simulink model "GuytonModel1986All_R2015a"  (R2015a)
settings: Solver=ode15s  StartTime=0  StopTime=383040  FixedStep=0.03  MaxStep=360  RelTol=1e-3
libraries: simulink x3
(part 2 of 5)

== system GuytonModel1986All_R2015a/Afferent Arteriole ==
  note: AFFERENT ARTERIOLE
  note: RNAUG1
  note: AUMK
  AARK : Inport
  MYOGRSAA : Inport  Port=2
  RNAUG1 : Inport  Port=3
  ANM : Inport  Port=4
  AUM : Inport  Port=5
  VIM : Inport  Port=6
  ANMAM : Constant  Value=0.5
  ANMAM1 : Constant
  ANMAM2 : Constant
  ARF : Constant  Value=1.5
  Constant1 : Constant
  Constant35 : Constant
  Product1 : Product  SaturateOnIntegerOverflow=on  RndMeth=Zero  InputSameDT=on  OutDataTypeStr=Inherit: Same as first input
  Product11 : Product  SaturateOnIntegerOverflow=on  RndMeth=Zero  InputSameDT=on  OutDataTypeStr=Inherit: Same as first input
  Product12 : Product  Inputs=6  SaturateOnIntegerOverflow=on  RndMeth=Zero  InputSameDT=on  OutDataTypeStr=Inherit: Same as first input
  Sum1 : Sum  SaturateOnIntegerOverflow=on  InputSameDT=on  OutDataTypeStr=Inherit: Same as first input
  Sum18 : Sum  Inputs=+-  SaturateOnIntegerOverflow=on  InputSameDT=on  OutDataTypeStr=Inherit: Same as first input
  Sum2 : Sum  Inputs=+-  SaturateOnIntegerOverflow=on  InputSameDT=on  OutDataTypeStr=Inherit: Same as first input
  Sum3 : Sum  SaturateOnIntegerOverflow=on  InputSameDT=on  OutDataTypeStr=Inherit: Same as first input
  lower limit 0.8 : Saturate  UpperLimit=inf  LowerLimit=0.86
  lower limit 0.86 : Saturate  UpperLimit=inf  LowerLimit=0.86
  lower limit 18 : Saturate  UpperLimit=inf  LowerLimit=18
  AAR : Outport
  wires:
  ANM/1 -> Sum18/1
  Constant35/1 -> Sum18/2
  ANMAM/1 -> Product11/2
  Sum18/1 -> Product11/1
  Product12/1 -> lower limit 18/1
  lower limit 18/1 -> AAR/1
  Product11/1 -> Sum1/1
  ANMAM1/1 -> Sum1/2
  Sum1/1 -> lower limit 0.86/1
  AARK/1 -> Product12/1  "AARK"
  MYOGRSAA/1 -> Product12/2  "MYOGRSAA"
  RNAUG1/1 -> Product12/3
  VIM/1 -> Product12/4  "VIM"
  lower limit 0.86/1 -> Product12/6  "ANIM"
  AUM/1 -> Sum2/1
  Constant1/1 -> Sum2/2
  Sum2/1 -> Product1/1
  ARF/1 -> Product1/2
  Product1/1 -> Sum3/1
  ANMAM2/1 -> Sum3/2
  Sum3/1 -> lower limit 0.8/1
  lower limit 0.8/1 -> Product12/5

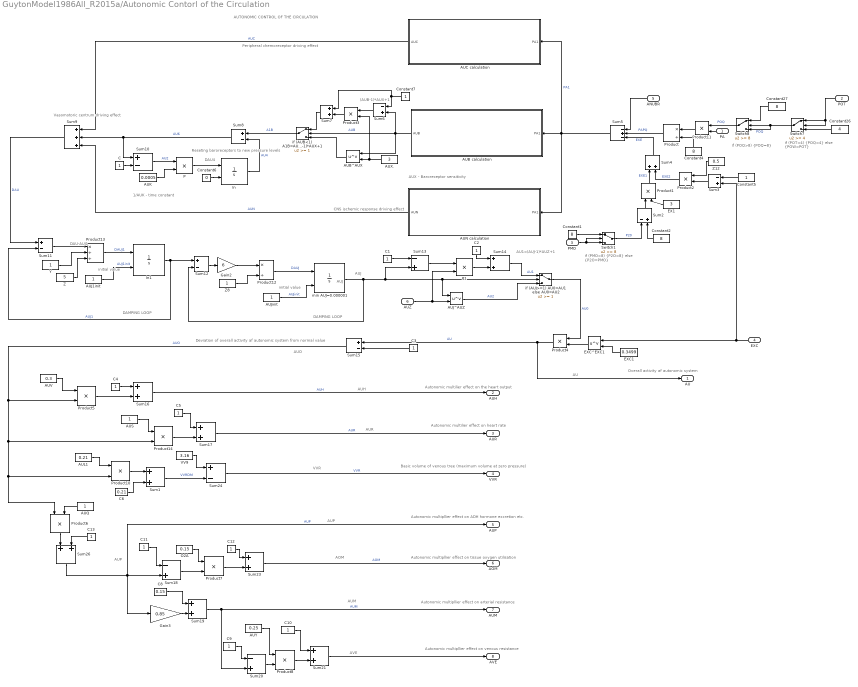
== system GuytonModel1986All_R2015a/Autonomic Contorl of the Circulation ==
  note: AUTONOMIC CONTROL OF THE CIRCULATION
  note: Autonomic multipllier effect on venous resistance
  note: Autonomic multipllier effect on arterial resistance
  note: Basic volume of venous tree (maximum volume at zero pressure)
  note: Autonomic multilier effect on heart rate
  note: Autonomic multipllier effect on tissue oxygen utilisation
  note: Autonomic multipllier effect on ADH hormone excretion etc.
  note: Autonomic multilier effect on the heart output
  note: Deviation of overall activity af autonomic system from normal value
  note: AUO
  note: Overall activity af autonomic system
  note: AU
  note: AU1=(AUJ-1)*AUZ+1
  note: initial value
  note: AUJ
  note: DAMPING LOOP
  note: DAMPING LOOP
  note: initial value
  note: AUJ
  note: DAU-AUJ1
  note: 1/AUK - time constant
  note: CNS ischemic response driving effect
  note: Vasomotoric centrum driving effect
  note: Peripheral chemoreceptor driving effect
  note: Reseting baroreceptors to new pressure levels
  note: DAU4
  note: AUX - Baroreceptor sensitivity
  note: (AUB-1)*AUX+1
  note: if (PMO>8)  {P2O=8}
      | else {P2O=PMO}
  note: if (POQ>8) {POQ=8}
  note: if (POT<4) {POQ=4}
      | else {POW=POT}
  note: AOM
  note: AUP
  note: AVE
  note: AUM
  note: VVR
  note: AUP
  note: AUR
  note: AUH
  PA : Inport
  POT : Inport  Port=2
  PMO : Inport  Port=3
  EXC : Inport  Port=4
  ANUBR : Inport  Port=5
  AUZ : Inport  Port=6
  AUB calculation : Subsystem
      mask Display: disp('AUB CALCULATION \n\nwhen PA1<40: AUB=1.85718             \nwhen  40>PA1<170: AUB=0.014286*(170-PA1)\nwhen PA1>=170: AUB=0               \n')
  AUB^AUX : Math  Operator=pow  SaturateOnIntegerOverflow=on
  AUC calculation : Subsystem
      mask Display: disp('AUC CALCULATION \n\nwhen PA1<40: AUC=1.2             \nwhen  40>PA1<80: AUC=0.03*(80-PA1)\nwhen PA1>=80: AUC=0               \n')
  AUJ1init : Constant
  AUJ^AUZ : Math  Operator=pow  SaturateOnIntegerOverflow=on
  AUJinit : Constant
  AUK : Constant  Value=0.0005
  AUL1 : Constant  Value=0.21
  AUN calculation : Subsystem
      mask Display: disp('AUN CALCULATION \n\nwhen PA1<50: AUN=6             \nwhen  20>PA1<50: AUN=0.2*(50-PA1)\nwhen PA1>=50: AUC=0               \n')
  AUQ : Constant
  AUS : Constant
  AUV : Constant  Value=0.3
  AUX. : Constant  Value=3
  AUY : Constant  Value=0.25
  C{,1..5,9..13} (11 alike) : Constant
  C6 : Constant  Value=0.21
  C8 : Constant  Value=0.15
  Constant{1..2,4,27} (4 alike) : Constant  Value=8
  Constant26 : Constant  Value=4
  Constant5 : Constant
  Constant6 : Constant  Value=0
  Constant7 : Constant
  EX1 : Constant  Value=3
  EXC1 : Constant  Value=0.3499
  EXC^EXC1 : Math  Operator=pow  SaturateOnIntegerOverflow=on
  Gain2 : Gain  Gain=6  SaturateOnIntegerOverflow=on  OutDataTypeStr=Inherit: Same as input  ParamDataTypeStr=Inherit: Same as input
  Gain3 : Gain  Gain=0.85  SaturateOnIntegerOverflow=on  OutDataTypeStr=Inherit: Same as input  ParamDataTypeStr=Inherit: Same as input
  In : Integrator  InitialConditionSource=external  InitialCondition=0.012127
  In1 : Integrator  InitialConditionSource=external  InitialCondition=1
  O2A : Constant  Value=0.15
  P : Product  SaturateOnIntegerOverflow=on  RndMeth=Zero  InputSameDT=on  OutDataTypeStr=Inherit: Same as first input
  P1 : Product  SaturateOnIntegerOverflow=on  RndMeth=Zero  InputSameDT=on  OutDataTypeStr=Inherit: Same as first input
  Product : Product  Inputs=*/  SaturateOnIntegerOverflow=on  RndMeth=Zero  InputSameDT=on  OutDataTypeStr=Inherit: Same as first input
  Product{1..8,10..11,14} (11 alike) : Product  SaturateOnIntegerOverflow=on  RndMeth=Zero  InputSameDT=on  OutDataTypeStr=Inherit: Same as first input
  Product12 : Product  Inputs=*/  SaturateOnIntegerOverflow=on  RndMeth=Zero  InputSameDT=on  OutDataTypeStr=Inherit: Same as first input
  Product13 : Product  Inputs=*//  SaturateOnIntegerOverflow=on  RndMeth=Zero  InputSameDT=on  OutDataTypeStr=Inherit: Same as first input
  Sum{1,4,7,14,16..17,19,21,23,26} (10 alike) : Sum  SaturateOnIntegerOverflow=on  InputSameDT=on  OutDataTypeStr=Inherit: Same as first input
  Sum{8,10..12,15,24} (6 alike) : Sum  Inputs=+-  SaturateOnIntegerOverflow=on  InputSameDT=on  OutDataTypeStr=Inherit: Same as first input
  Sum{2..3,6,13,18,20} (6 alike) : Sum  Inputs=-+  SaturateOnIntegerOverflow=on  InputSameDT=on  OutDataTypeStr=Inherit: Same as first input
  Sum5 : Sum  Inputs=-+-  SaturateOnIntegerOverflow=on  InputSameDT=on  OutDataTypeStr=Inherit: Same as first input
  Sum9 : Sum  Inputs=+++  SaturateOnIntegerOverflow=on  InputSameDT=on  OutDataTypeStr=Inherit: Same as first input
  Switch1 : Switch  Threshold=8  SaturateOnIntegerOverflow=on  InputSameDT=on
  Switch7 : Switch  Threshold=4  SaturateOnIntegerOverflow=on  InputSameDT=on
  Switch8 : Switch  Threshold=8  SaturateOnIntegerOverflow=on  InputSameDT=on
  VV9 : Constant  Value=3.16
  Y : Constant
  Z : Constant  Value=5
  Z12 : Constant  Value=0.5
  Z8 : Constant
  if (AUB<1) A1B=AUB^AUX else A1B=(AUB-1)*AUX+1 : Switch  Threshold=1  SaturateOnIntegerOverflow=on  InputSameDT=on
  if (AUJ>=1) AU0=AU1 else AU0=AU2 : Switch  Threshold=1  SaturateOnIntegerOverflow=on  InputSameDT=on
  min AUJ=0.000001 : Integrator  InitialConditionSource=external  InitialCondition=1  LimitOutput=on  LowerSaturationLimit=0
  AU : Outport
  AUH : Outport  Port=2
  AUR : Outport  Port=3
  VVR : Outport  Port=4
  AUP : Outport  Port=5
  AOM : Outport  Port=6
  AUM : Outport  Port=7
  AVE : Outport  Port=8
  wires:
  Constant6/1 -> In/2
  Sum21/1 -> AVE/1
  C10/1 -> Sum21/1
  Product8/1 -> Sum21/2
  AUY/1 -> Product8/1
  Sum20/1 -> Product8/2
  Sum1/1 -> Sum24/2  "VVRDM"
  Product10/1 -> Sum1/1
  C6/1 -> Sum1/2
  Sum24/1 -> VVR/1  "VVR"
  VV9/1 -> Sum24/1
  AUL1/1 -> Product10/1
  C13/1 -> Sum26/2
  Product6/1 -> Sum26/1
  EXC^EXC1/1 -> Product4/2
  EXC1/1 -> EXC^EXC1/2
  C1/1 -> Sum13/1
  Sum13/1 -> P1/1
  AUJinit/1 -> min AUJ=0.000001/2  "AUJinit"
  AUJ1init/1 -> In1/2  "AUJ1init"
  In1/1 -> Sum11/2, Sum12/1  "AUJ1"
  AUX./1 -> Product3/2, AUB^AUX/2
  AUB^AUX/1 -> if (AUB<1) A1B=AUB^AUX else A1B=(AUB-1)*AUX+1/3
  Sum7/1 -> if (AUB<1) A1B=AUB^AUX else A1B=(AUB-1)*AUX+1/1
  Product3/1 -> Sum7/2
  Sum6/1 -> Product3/1
  Constant7/1 -> Sum6/1, Sum7/1
  AUB calculation/1(AUB) -> AUB^AUX/1, Sum6/2, if (AUB<1) A1B=AUB^AUX else A1B=(AUB-1)*AUX+1/2  "AUB"
  Switch1/1 -> Sum2/1  "P20"
  PMO/1 -> Switch1/3, Switch1/2
  Constant1/1 -> Switch1/1
  EXC/1 -> EXC^EXC1/1, Sum3/2
  Switch8/1 -> Product11/1  "POQ"
  Constant27/1 -> Switch8/1
  Switch7/1 -> Switch8/3, Switch8/2  "POQ"
  Constant26/1 -> Switch7/3
  Product11/1 -> Product/1
  Product/1 -> Sum5/2  "PAPQ"
  C12/1 -> Sum23/1
  Product7/1 -> Sum23/2
  O2A/1 -> Product7/1
  Sum18/1 -> Product7/2
  C11/1 -> Sum18/1
  Sum19/1 -> AUM/1, Sum20/2  "AUM"
  C9/1 -> Sum20/1
  C8/1 -> Sum19/1
  Gain3/1 -> Sum19/2
  Sum26/1 -> Gain3/1, Sum18/2, AUP/1  "AUP"
  AUQ/1 -> Product6/2
  Sum17/1 -> AUR/1  "AUR"
  C5/1 -> Sum17/1
  Product14/1 -> Sum17/2
  AUS/1 -> Product14/1
  C4/1 -> Sum16/1
  Product5/1 -> Sum16/2
  AUV/1 -> Product5/1
  C3/1 -> Sum15/2
  Product4/1 -> Sum15/1, AU/1  "AU"
  Sum14/1 -> if (AUJ>=1) AU0=AU1 else AU0=AU2/1  "AU1"
  C2/1 -> Sum14/1
  P1/1 -> Sum14/2
  AUJ^AUZ/1 -> if (AUJ>=1) AU0=AU1 else AU0=AU2/3  "AU2"
  min AUJ=0.000001/1 -> Sum12/2, AUJ^AUZ/1, if (AUJ>=1) AU0=AU1 else AU0=AU2/2, Sum13/2
  Product12/1 -> min AUJ=0.000001/1  "DAUJ"
  Gain2/1 -> Product12/1
  Sum12/1 -> Gain2/1
  Y/1 -> Product13/2
  P/1 -> In/1
  AUK/1 -> P/2
  Sum10/1 -> P/1  "AU2"
  C/1 -> Sum10/2
  Sum8/1 -> Sum9/2, Sum10/1  "AU6"
  ANUBR/1 -> Sum5/1
  Product1/1 -> Sum4/1  "EXE1"
  Product2/1 -> Sum4/2  "EXE2"
  Z12/1 -> Product2/1
  Sum3/1 -> Product2/2
  Constant5/1 -> Sum3/1
  EX1/1 -> Product1/2
  Sum2/1 -> Product1/1
  Constant2/1 -> Sum2/2
  AUZ/1 -> P1/2, AUJ^AUZ/2
  Sum4/1 -> Sum5/3  "EXE"
  POT/1 -> Switch7/1, Switch7/2
  Constant4/1 -> Product/2
  PA/1 -> Product11/2
  Sum5/1 -> AUN calculation/1(PA1), AUB calculation/1(PA1), AUC calculation/1(PA1)  "PA1"
  AUN calculation/1(AUN) -> Sum9/3  "AUN"
  AUC calculation/1(AUC) -> Sum9/1  "AUC"
  if (AUB<1) A1B=AUB^AUX else A1B=(AUB-1)*AUX+1/1 -> Sum8/1  "A1B"
  In/1 -> Sum8/2  "AU4"
  Sum9/1 -> Sum11/1  "DAU"
  Z/1 -> Product13/3
  Product13/1 -> In1/1  "DAUJ1"
  Sum11/1 -> Product13/1
  Z8/1 -> Product12/2
  if (AUJ>=1) AU0=AU1 else AU0=AU2/1 -> Product4/1  "AU0"
  Sum15/1 -> Product10/2, Product6/1, Product14/2, Product5/2  "AUO"
  Sum23/1 -> AOM/1  "AOM"
  Sum16/1 -> AUH/1  "AUH"

== system GuytonModel1986All_R2015a/Blood viscosity ==
  note: HM
  note: VIM
  note: Blood viscosity
  HM : Inport
  Constant1 : Constant  Value=3
  Constant7 : Constant  Value=1.5
  HKM : Constant  Value=0.53333
  HMK : Constant  Value=90
  Product1 : Product  Inputs=*/  SaturateOnIntegerOverflow=on  RndMeth=Zero  InputSameDT=on  OutDataTypeStr=Inherit: Same as first input
  Product7 : Product  Inputs=*/  SaturateOnIntegerOverflow=on  RndMeth=Zero  InputSameDT=on  OutDataTypeStr=Inherit: Same as first input
  Product8 : Product  Inputs=*/  SaturateOnIntegerOverflow=on  RndMeth=Zero  InputSameDT=on  OutDataTypeStr=Inherit: Same as first input
  Sum8 : Sum  Inputs=+-  SaturateOnIntegerOverflow=on  InputSameDT=on  OutDataTypeStr=Inherit: Same as first input
  Sum9 : Sum  SaturateOnIntegerOverflow=on  InputSameDT=on  OutDataTypeStr=Inherit: Same as first input
  VIM : Outport
  wires:
  Constant1/1 -> Product1/2
  Product1/1 -> VIM/1
  HM/1 -> Product7/1, Sum8/2  "HM"
  HMK/1 -> Sum8/1
  Sum8/1 -> Product7/2
  Product7/1 -> Product8/1
  HKM/1 -> Product8/2
  Product8/1 -> Sum9/1  "VIE"
  Constant7/1 -> Sum9/2
  Sum9/1 -> Product1/1  "VIB"

== system GuytonModel1986All_R2015a/Capillary Membrane Fluid Dynamics ==
  note: Capillary Membrane Fluid Dynamics
  PC : Inport
  PPC : Inport  Port=2
  PGH : Inport  Port=3
  PTC : Inport  Port=4
  VTL : Inport  Port=5
  TVD : Inport  Port=6
  VUD : Inport  Port=7
  DFP : Inport  Port=8
  VID : Inport  Port=9
  CFC : Inport  Port=10
  VPN : Inport  Port=11
  VTSN : Inport  Port=12
  Add : Sum
  Add1 : Sum  Inputs=-+
  CPK : Constant  Value=0.000253
  Integrator : Integrator  InitialConditionSource=external
  Integrator1 : Integrator  InitialConditionSource=external
  Math Function : Math  Operator=pow  SaturateOnIntegerOverflow=on
  PCE : Constant  Value=1.000
  PCR : Constant  Value=15
  PCR1 : Constant  Value=0
  Product : Product  RndMeth=Zero
  Product1 : Product  RndMeth=Zero
  Product2 : Product  Inputs=*/  RndMeth=Zero
  Product3 : Product  Inputs=*/  RndMeth=Zero
  Sum1 : Sum  Inputs=-++--  SaturateOnIntegerOverflow=on  InputSameDT=on  OutDataTypeStr=Inherit: Same as first input
  Sum2 : Sum  Inputs=-+-  SaturateOnIntegerOverflow=on  InputSameDT=on  OutDataTypeStr=Inherit: Same as first input
  Sum3 : Sum  Inputs=+--+  SaturateOnIntegerOverflow=on  InputSameDT=on  OutDataTypeStr=Inherit: Same as first input
  "if (PCRD1<0)  {PCRD=0} else {PCRD=PCRD1}" : Switch
  VP : Outport
  VTCLP : Outport  Port=2
  VTS : Outport  Port=3
  CFILTR : Outport  Port=4
  VTC : Outport  Port=5
  VPREL : Outport  Port=6
  VTSREL : Outport  Port=7
  wires:
  PC/1 -> Sum3/1, Add1/2
  PPC/1 -> Sum3/2
  PGH/1 -> Sum3/3
  PTC/1 -> Sum3/4
  Sum3/1 -> Product/1  "PCGR"
  CFC/1 -> Product/2
  Product/1 -> Add/2, CFILTR/1  "CFILTR"
  PCR/1 -> Add1/1
  Add1/1 -> "if (PCRD1<0)  {PCRD=0} else {PCRD=PCRD1}"/2, "if (PCRD1<0)  {PCRD=0} else {PCRD=PCRD1}"/1  "PCRD1"
  PCR1/1 -> "if (PCRD1<0)  {PCRD=0} else {PCRD=PCRD1}"/3
  "if (PCRD1<0)  {PCRD=0} else {PCRD=PCRD1}"/1 -> Product1/2  "PCRD"
  CPK/1 -> Product1/1
  Math Function/1 -> Add/1, VTCLP/1  "VTCPL"
  Add/1 -> Sum2/2, Sum1/1, VTC/1  "VTC"
  VTL/1 -> Sum1/2, Sum2/1
  TVD/1 -> Sum1/3
  VUD/1 -> Sum1/4
  DFP/1 -> Sum1/5
  Sum1/1 -> Integrator/1  "VPD"
  VTSN/1 -> Integrator1/2, Product3/2
  Sum2/1 -> Integrator1/1  "VTS"
  VID/1 -> Sum2/3
  Integrator/1 -> VP/1, Product2/1  "VP"
  Integrator1/1 -> VTS/1, Product3/1  "VTS"
  Product1/1 -> Math Function/1  "U"
  PCE/1 -> Math Function/2  "v"
  VPN/1 -> Integrator/2, Product2/2
  Product2/1 -> VPREL/1
  Product3/1 -> VTSREL/1

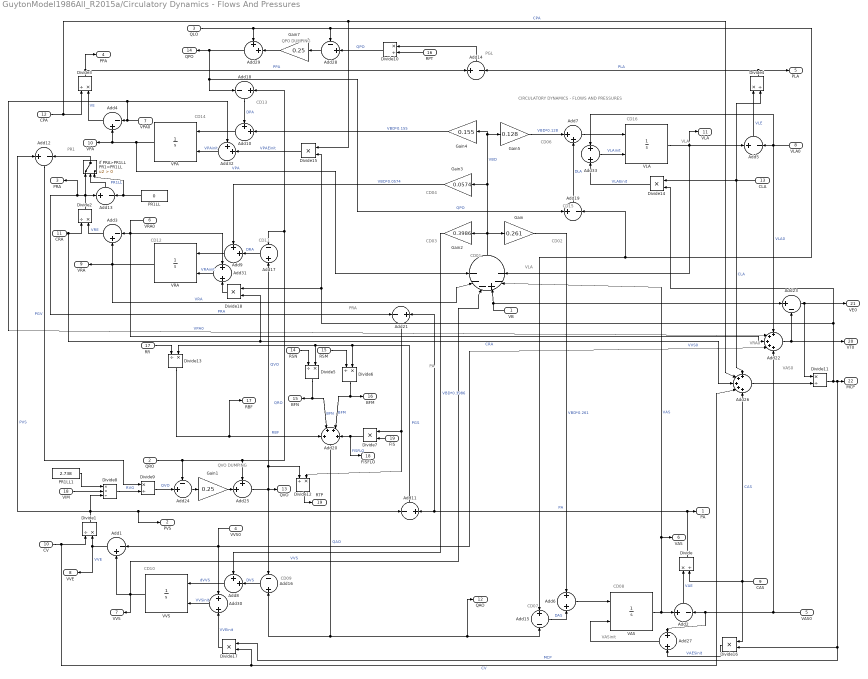
== system GuytonModel1986All_R2015a/Circulatory Dynamics - Flows And Pressures ==
  note: CD16
  note: CD15
  note: CD14
  note: CD12
  note: CD11
  note: CD10
  note: CD09
  note: CD08
  note: CD07
  note: CD06
  note: CD13
  note: CD04
  note: CD03
  note: CD02
  note: CD01
  note: CIRCULATORY DYNAMICS - FLOWS AND PRESSURES
  note: VAS0
  note: VRA0
  note: VASinit
  note: PRA
  note: PA
  note: PGL
  note: PR1
  note: VLA
  note: VLA
  note: QVO DUMPING
  note: QPO DUMPING
  VB : Inport
  QRO : Inport  Port=2
  QLO : Inport  Port=3
  VVS0 : Inport  Port=4
  VAS0 : Inport  Port=5
  VRA0 : Inport  Port=6
  VPA0 : Inport  Port=7
  VLA0 : Inport  Port=8
  CAS : Inport  Port=9
  CV : Inport  Port=10
  CRA : Inport  Port=11
  CPA : Inport  Port=12
  CLA : Inport  Port=13
  RSN : Inport  Port=14
  RSM : Inport  Port=15
  RPT : Inport  Port=16
  RR : Inport  Port=17
  VIM : Inport  Port=18
  FIS : Inport  Port=19
  " " : Sum  Inputs=---+--
  " VAS" : Integrator  InitialConditionSource=external
  " VLA" : Integrator  InitialConditionSource=external
  " VPA" : Integrator  InitialConditionSource=external
  " VRA" : Integrator  InitialConditionSource=external
  " VVS" : Integrator  InitialConditionSource=external
  Add1 : Sum  Inputs=|-+
  Add{8..10,25,29,32} (6 alike) : Sum  Inputs=++|
  Add{11,16..18,21} (5 alike) : Sum  Inputs=-+
  Add{2,5,12..15,19} (7 alike) : Sum  Inputs=+-
  Add20 : Sum  Inputs=++++
  Add22 : Sum  Inputs=5
  Add23 : Sum  Inputs=|+-
  Add24 : Sum  Inputs=-+|
  Add26 : Sum  Inputs=5
  Add{6,27,30..31,33} (5 alike) : Sum
  Add28 : Sum  Inputs=-+|
  Add3 : Sum  Inputs=|-+
  Add4 : Sum  Inputs=|-+
  Add7 : Sum  Inputs=|++
  Divide{,4,9..11} (5 alike) : Product  Inputs=*/
  Divide{1..3,5..6,12..13} (7 alike) : Product  Inputs=/*
  Divide{7,14..18} (6 alike) : Product  Inputs=**
  Divide8 : Product  Inputs=**/
  Gain : Gain  Gain=0.261
  Gain1 : Gain  Gain=0.25
  Gain2 : Gain  Gain=0.3986
  Gain3 : Gain  Gain=0.0574
  Gain4 : Gain  Gain=0.155
  Gain5 : Gain  Gain=0.128
  Gain7 : Gain  Gain=0.25
  PR1LL : Constant  Value=0
  PR1LL1 : Constant  Value=2.738
  if PRA>PR1LL PR1=PR1LL : Switch  Criteria=u2 > Threshold
  PA : Outport
  PVS : Outport  Port=2
  PRA : Outport  Port=3
  PPA : Outport  Port=4
  PLA : Outport  Port=5
  VAS : Outport  Port=6
  VVS : Outport  Port=7
  VVE : Outport  Port=8
  VRA : Outport  Port=9
  VPA : Outport  Port=10
  VLA : Outport  Port=11
  QAO : Outport  Port=12
  QVO : Outport  Port=13
  QPO : Outport  Port=14
  BFN : Outport  Port=15
  BFM : Outport  Port=16
  RBF : Outport  Port=17
  FISFLO : Outport  Port=18
  RTP : Outport  Port=19
  VT0 : Outport  Port=20
  VE0 : Outport  Port=21
  MCP : Outport  Port=22
  wires:
  Add33/1 -> " VLA"/2  "VLAinit"
  Divide15/1 -> Add32/2  "VPAEinit"
  Add32/1 -> " VPA"/2  "VPAinit"
  Divide18/1 -> Add31/2
  Add31/1 -> " VRA"/2  "VRAinit"
  Divide17/1 -> Add30/2  "VVEinit"
  Add30/1 -> " VVS"/2  "VVSinit"
  VVS0/1 -> Add22/4, Add1/1, Add30/1  "VVS0"
  Add27/1 -> " VAS"/2
  Divide16/1 -> Add27/2  "VAESinit"
  Divide14/1 -> Add33/2  "VLAEinit"
  Divide11/1 -> Divide17/1, Divide16/2, MCP/1, Divide15/2, Divide18/1, Divide14/2  "MCP"
  Add26/1 -> Divide11/2
  Divide13/1 -> Add20/1, RBF/1  "RBF"
  RR/1 -> Divide13/1
  Add6/1 -> " VAS"/1
  " "/1 -> Gain5/1, Gain4/1, Gain3/1, Gain2/1, Gain/1  "VBD"
  Add23/1 -> Divide11/1, VE0/1
  Add22/1 -> Add23/2, VT0/1
  if PRA>PR1LL PR1=PR1LL/1 -> Add12/2
  Add5/1 -> Divide4/1  "VLE"
  Add4/1 -> Divide3/2  "VE"
  Divide12/1 -> RTP/1
  Add11/1 -> Divide13/2, Divide5/2, Divide6/2  "PGS"
  RPT/1 -> Divide10/2
  Divide8/1 -> Divide9/2  "RVG"
  PR1LL1/1 -> Divide8/1
  VIM/1 -> Divide8/2
  Add20/1 -> QAO/1, Add15/2, Add16/2  "QAO"
  Divide9/1 -> Add24/2  "QVO"
  FIS/1 -> Divide7/2
  Add21/1 -> Divide7/1, Divide12/2
  Divide7/1 -> FISFLO/1, Add20/4  "FISFLO"
  Divide6/1 -> BFM/1, Add20/3  "BFM"
  RSM/1 -> Divide6/1
  Divide5/1 -> BFN/1, Add20/2  "BFN"
  RSN/1 -> Divide5/1
  QLO/1 -> Add19/2, Add15/1, Add28/1, Add29/1
  Add19/1 -> Add7/2  "DLA"
  Add18/1 -> Add10/1  "DPA"
  QRO/1 -> Add24/1, Add25/1, Add17/1, Add18/2  "QRO"
  Add17/1 -> Add9/2  "DRA"
  Add16/1 -> Add8/2  "DVS"
  Add15/1 -> Add6/2  "DAS"
  Add14/1 -> Divide10/1
  Divide3/1 -> PPA/1, Add14/1  "PPA"
  Add12/1 -> Divide9/1  "PGV"
  Add13/1 -> if PRA>PR1LL PR1=PR1LL/2
  PR1LL/1 -> if PRA>PR1LL PR1=PR1LL/3, Add13/2  "PR1LL"
  Divide2/1 -> Add21/1, PRA/1, Add13/1, if PRA>PR1LL PR1=PR1LL/1  "PRA"
  Divide1/1 -> Add12/1, PVS/1, Add11/1, Divide8/3  "PVS"
  CLA/1 -> Divide14/1, Add26/1, Divide4/2  "CLA"
  CV/1 -> Divide17/2, Add26/4, Divide1/1  "CV"
  CRA/1 -> Divide18/2, Add26/3, Divide2/1  "CRA"
  CPA/1 -> Divide15/1, Add26/2, Divide3/1  "CPA"
  VLA0/1 -> Add33/1, Add22/1, Add5/2  "VLA0"
  VRA0/1 -> Add22/3, Add3/1, Add31/1
  VPA0/1 -> Add4/1, Add32/1, Add22/2  "VPA0"
  Gain4/1 -> Add10/2  "VBD*0.155"
  Add10/1 -> " VPA"/1
  Add9/1 -> " VRA"/1
  Gain3/1 -> Add9/1  "VBD*0.0574"
  Add8/1 -> " VVS"/1  "dVVS"
  Gain2/1 -> Add8/1  "VBD*0.3986"
  " VPA"/1 -> VPA/1, Add4/2, " "/1  "VPA"
  " VRA"/1 -> Add3/2, " "/2, VRA/1  "VRA"
  Add3/1 -> Divide2/2  "VRE"
  Add1/1 -> Divide1/2, VVE/1  "VVE"
  " VVS"/1 -> " "/3, VVS/1, Add1/2  "VVS"
  Add7/1 -> " VLA"/1
  Gain5/1 -> Add7/1  "VBD*0.128"
  Gain/1 -> Add6/1  "VBD*0.261"
  VB/1 -> Add23/1, " "/4
  " VLA"/1 -> " "/6, VLA/1, Add5/1
  Divide4/1 -> PLA/1, Add14/2  "PLA"
  Divide/1 -> PA/1, Add11/2, Add21/2  "PA"
  CAS/1 -> Divide16/1, Divide/2, Add26/5  "CAS"
  Add2/1 -> Divide/1  "VAE"
  " VAS"/1 -> " "/5, VAS/1, Add2/1  "VAS"
  VAS0/1 -> Add27/1, Add2/2, Add22/5
  Gain1/1 -> Add25/2
  Add25/1 -> Divide12/1, Add17/2, Add16/1, QVO/1  "QVO"
  Add24/1 -> Gain1/1
  Add29/1 -> QPO/1, Add19/1, Add18/1  "QPO"
  Divide10/1 -> Add28/2  "QPO"
  Add28/1 -> Gain7/1
  Gain7/1 -> Add29/2

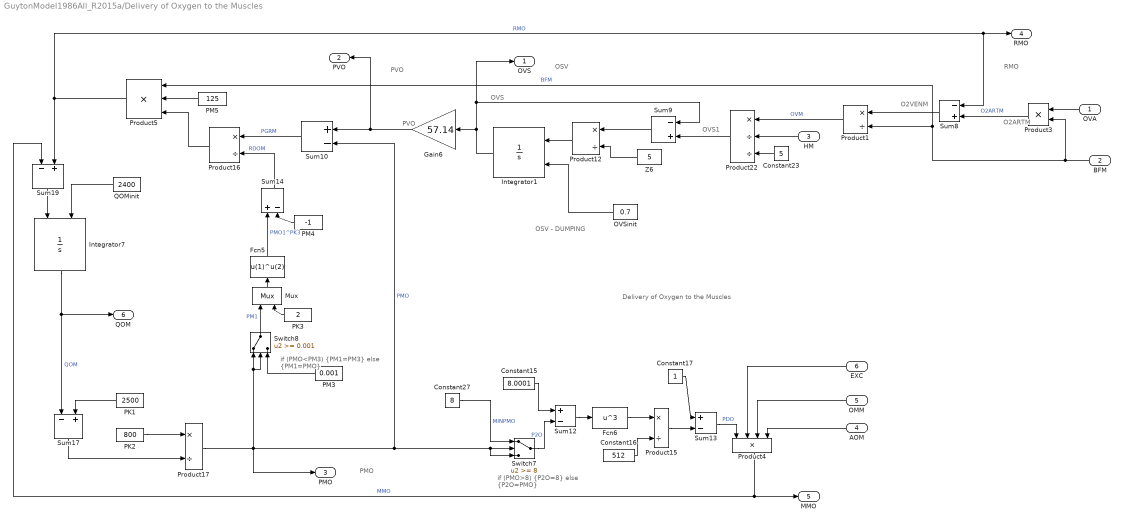
== system GuytonModel1986All_R2015a/Delivery of Oxygen to the Muscles  ==
  note: if (PMO>8)  {P2O=8}
      | else {P2O=PMO}
  note: if (PMO<PM3) {PM1=PM3}
      | else {PM1=PMO}
  note: OSV - DUMPING
  note: OSV
  note: PVO
  note: OVS
  note: OVS1
  note: O2VENM
  note: O2ARTM
  note: RMO
  note: PMO
  note: PVO
  note: Delivery of Oxygen to the Muscles
  OVA : Inport
  BFM : Inport  Port=2
  HM : Inport  Port=3
  AOM : Inport  Port=4
  OMM : Inport  Port=5
  EXC : Inport  Port=6
  Constant15 : Constant  Value=8.0001
  Constant16 : Constant  Value=512
  Constant17 : Constant
  Constant23 : Constant  Value=5
  Constant27 : Constant  Value=8
  Fcn5 : Fcn  Expr=u(1)^u(2)
  Fcn6 : Fcn  Expr=u^3
  Gain6 : Gain  Gain=57.14  SaturateOnIntegerOverflow=on  OutDataTypeStr=Inherit: Same as input  ParamDataTypeStr=Inherit: Same as input
  Integrator1 : Integrator  InitialConditionSource=external  InitialCondition=0.6855
  Integrator7 : Integrator  InitialConditionSource=external  InitialCondition=2399.9633789
  Mux : Mux  Inputs=2
  OVSinit : Constant  Value=0.7
  PK1 : Constant  Value=2500
  PK2 : Constant  Value=800
  PK3 : Constant  Value=2
  PM3 : Constant  Value=0.001
  PM4 : Constant  Value=-1
  PM5 : Constant  Value=125
  Product{1,12,15..17} (5 alike) : Product  Inputs=*/  SaturateOnIntegerOverflow=on  RndMeth=Zero  InputSameDT=on  OutDataTypeStr=Inherit: Same as first input
  Product22 : Product  Inputs=*//  SaturateOnIntegerOverflow=on  RndMeth=Zero  InputSameDT=on  OutDataTypeStr=Inherit: Same as first input
  Product3 : Product  SaturateOnIntegerOverflow=on  RndMeth=Zero  InputSameDT=on  OutDataTypeStr=Inherit: Same as first input
  Product4 : Product  Inputs=4  SaturateOnIntegerOverflow=on  RndMeth=Zero  InputSameDT=on  OutDataTypeStr=Inherit: Same as first input
  Product5 : Product  Inputs=3  SaturateOnIntegerOverflow=on  RndMeth=Zero  InputSameDT=on  OutDataTypeStr=Inherit: Same as first input
  QOMinit : Constant  Value=2400
  Sum{10,12..14} (4 alike) : Sum  Inputs=+-  SaturateOnIntegerOverflow=on  InputSameDT=on  OutDataTypeStr=Inherit: Same as first input
  Sum{8..9,17,19} (4 alike) : Sum  Inputs=-+  SaturateOnIntegerOverflow=on  InputSameDT=on  OutDataTypeStr=Inherit: Same as first input
  Switch7 : Switch  Threshold=8  SaturateOnIntegerOverflow=on  InputSameDT=on
  Switch8 : Switch  Threshold=0.001  SaturateOnIntegerOverflow=on  InputSameDT=on
  Z6 : Constant  Value=5
  OVS : Outport
  PVO : Outport  Port=2
  PMO : Outport  Port=3
  RMO : Outport  Port=4
  MMO : Outport  Port=5
  QOM : Outport  Port=6
  wires:
  Constant27/1 -> Switch7/1  "MINPMO"
  QOMinit/1 -> Integrator7/2
  Product5/1 -> Sum8/1, RMO/1, Sum19/2  "RMO"
  PM5/1 -> Product5/2
  Product16/1 -> Product5/3
  Sum10/1 -> Product16/1  "PGRM"
  OVSinit/1 -> Integrator1/2
  Constant23/1 -> Product22/3
  HM/1 -> Product22/2
  Product1/1 -> Product22/1  "OVM"
  Sum8/1 -> Product1/1
  PK3/1 -> Mux/2
  Switch8/1 -> Mux/1  "PM1"
  Mux/1 -> Fcn5/1
  AOM/1 -> Product4/4
  Product17/1 -> PMO/1, Switch7/3, Switch7/2, Sum10/2, Switch8/2, Switch8/1  "PMO"
  PM3/1 -> Switch8/3
  PK2/1 -> Product17/1
  PM4/1 -> Sum14/2
  Fcn5/1 -> Sum14/1  "PMO1^PK3"
  OMM/1 -> Product4/3
  EXC/1 -> Product4/2
  Sum13/1 -> Product4/1  "PDO"
  Constant17/1 -> Sum13/1
  Product15/1 -> Sum13/2
  Constant16/1 -> Product15/2
  Fcn6/1 -> Product15/1
  Sum12/1 -> Fcn6/1
  Constant15/1 -> Sum12/1
  Switch7/1 -> Sum12/2  "P2O"
  Gain6/1 -> PVO/1, Sum10/1
  Sum9/1 -> Product12/1
  Z6/1 -> Product12/2
  Product22/1 -> Sum9/2
  Product3/1 -> Sum8/2  "O2ARTM"
  OVA/1 -> Product3/1
  BFM/1 -> Product5/1, Product1/2, Product3/2  "BFM"
  Product12/1 -> Integrator1/1
  Integrator1/1 -> OVS/1, Sum9/1, Gain6/1
  Integrator7/1 -> QOM/1, Sum17/1  "QOM"
  PK1/1 -> Sum17/2
  Sum19/1 -> Integrator7/1
  Sum17/1 -> Product17/2
  Sum14/1 -> Product16/2  "RDOM"
  Product4/1 -> MMO/1, Sum19/1  "MMO"

== system GuytonModel1986All_R2015a/Delivery of Oxygen to the Non-muscleTtissues ==
  note: OSV
  note: if (POT>8)  {P1O=8}
      | else {P1O=PTO}
  note: if (P3<50) {RDO=50}
      | else {RDO=P3}
  note: P1O
  note: MO2
  note: OSV
  note: P3=POT^3
  note: PDO
  note: DAMPING
  note: OSV
  note: OVV
  note: DOB
  note: POT
  note: POV
  note: OSV - DUMPING
  note: Delivery of Oxygen to the Non-muscleTtissues
  OVA : Inport
  BFN : Inport  Port=2
  HM : Inport  Port=3
  AOM : Inport  Port=4
  O2M : Inport  Port=5
  Constant10 : Constant  Value=8.0001
  Constant11 : Constant  Value=512
  Constant12 : Constant
  Constant8 : Constant  Value=50
  Constant9 : Constant  Value=8
  DOBinit : Constant  Value=0.7
  Fcn3 : Fcn  Expr=u^3
  Gain3 : Gain  Gain=57.14  SaturateOnIntegerOverflow=on  OutDataTypeStr=Inherit: Same as input  ParamDataTypeStr=Inherit: Same as input
  Gain5 : Gain  Gain=0.00333  SaturateOnIntegerOverflow=on  OutDataTypeStr=Inherit: Same as input  ParamDataTypeStr=Inherit: Same as input
  Integrator QO2 : Integrator  InitialConditionSource=external  InitialCondition=2403.143066
  ONM4 : Constant  Value=5
  PN5 : Constant  Value=964
  POT^3 : Fcn  Expr=u^3
  Product{,4,6..7} (4 alike) : Product  Inputs=*/  SaturateOnIntegerOverflow=on  RndMeth=Zero  InputSameDT=on  OutDataTypeStr=Inherit: Same as first input
  Product1 : Product  SaturateOnIntegerOverflow=on  RndMeth=Zero  InputSameDT=on  OutDataTypeStr=Inherit: Same as first input
  Product2 : Product  Inputs=3  SaturateOnIntegerOverflow=on  RndMeth=Zero  InputSameDT=on  OutDataTypeStr=Inherit: Same as first input
  Product21 : Product  Inputs=*//  SaturateOnIntegerOverflow=on  RndMeth=Zero  InputSameDT=on  OutDataTypeStr=Inherit: Same as first input
  Product3 : Product  Inputs=3  SaturateOnIntegerOverflow=on  RndMeth=Zero  InputSameDT=on  OutDataTypeStr=Inherit: Same as first input
  Sum18 : Sum  Inputs=-+  SaturateOnIntegerOverflow=on  InputSameDT=on  OutDataTypeStr=Inherit: Same as first input
  Sum2 : Sum  Inputs=-+  SaturateOnIntegerOverflow=on  InputSameDT=on  OutDataTypeStr=Inherit: Same as first input
  Sum3 : Sum  Inputs=-+  SaturateOnIntegerOverflow=on  InputSameDT=on  OutDataTypeStr=Inherit: Same as first input
  Sum4 : Sum  Inputs=+-  SaturateOnIntegerOverflow=on  InputSameDT=on  OutDataTypeStr=Inherit: Same as first input
  Sum6 : Sum  Inputs=+-  SaturateOnIntegerOverflow=on  InputSameDT=on  OutDataTypeStr=Inherit: Same as first input
  Sum7 : Sum  Inputs=+-  SaturateOnIntegerOverflow=on  InputSameDT=on  OutDataTypeStr=Inherit: Same as first input
  Switch4 : Switch  Threshold=50  SaturateOnIntegerOverflow=on  InputSameDT=on
  Switch5 : Switch  Threshold=8  SaturateOnIntegerOverflow=on  InputSameDT=on
  Z2 : Constant  Value=2403
  Z7 : Constant  Value=5
  integrator OSV : Integrator  InitialConditionSource=external  InitialCondition=0.6577
  OSV : Outport
  POV : Outport  Port=2
  POT : Outport  Port=3
  DOB : Outport  Port=4
  MO2 : Outport  Port=5
  QO2 : Outport  Port=6
  wires:
  PN5/1 -> Product3/2
  Sum2/1 -> Product4/1  "O2VENN"
  O2M/1 -> Product2/3
  Z2/1 -> Integrator QO2/2
  Product/1 -> Product3/3
  Product3/1 -> Sum2/1, DOB/1, Sum18/2  "DOB"
  Sum4/1 -> Product/1  "PGRV"
  DOBinit/1 -> integrator OSV/2
  Product6/1 -> integrator OSV/1
  Product1/1 -> Sum2/2  "O2ART"
  AOM/1 -> Product2/2
  Sum7/1 -> Product2/1
  Constant12/1 -> Sum7/1
  Product7/1 -> Sum7/2
  Constant11/1 -> Product7/2
  Fcn3/1 -> Product7/1
  Sum6/1 -> Fcn3/1
  Constant10/1 -> Sum6/1
  Switch5/1 -> Sum6/2
  Constant9/1 -> Switch5/1  "MINPOT"
  Constant8/1 -> Switch4/3
  POT^3/1 -> Switch4/1, Switch4/2
  Gain3/1 -> POV/1, Sum4/1
  Sum3/1 -> Product6/1
  Z7/1 -> Product6/2
  OVA/1 -> Product1/1
  Integrator QO2/1 -> QO2/1, Gain5/1  "QO2"
  Sum18/1 -> Integrator QO2/1  "DO2N"
  Switch4/1 -> Product/2  "RDO"
  Product2/1 -> MO2/1, Sum18/1  "MO2"
  HM/1 -> Product21/2  "HM"
  BFN/1 -> Product3/1, Product4/2, Product1/2  "BFN"
  integrator OSV/1 -> OSV/1, Sum3/1, Gain3/1
  Product21/1 -> Sum3/2  "OSV1"
  Gain5/1 -> POT/1, Sum4/2, Switch5/3, Switch5/2, POT^3/1  "POT"
  Product4/1 -> Product21/1
  ONM4/1 -> Product21/3

== system GuytonModel1986All_R2015a/Effect of stress relaxation on basic venous volume ==
  note: Effect of stress relaxation on basic venous volume
  VVE : Inport
  " 2" : Constant  Value=0.3
  ISRK1 : Constant  Value=60
  Integrator1 : Integrator  InitialConditionSource=external
  Integrator2 : Integrator  InitialConditionSource=external
  RAPDel=RAP-RAPAdp : Sum  Inputs=+-  SaturateOnIntegerOverflow=on  InputSameDT=on  OutDataTypeStr=Inherit: Same as first input
  RAPDel=RAP-RAPAdp1 : Sum  Inputs=+-  SaturateOnIntegerOverflow=on  InputSameDT=on  OutDataTypeStr=Inherit: Same as first input
  RAPDel=RAP-RAPAdp2 : Sum  Inputs=+-  SaturateOnIntegerOverflow=on  InputSameDT=on  OutDataTypeStr=Inherit: Same as first input
  RAPdot=RAPdel/AffTau : Product  SaturateOnIntegerOverflow=on  InputSameDT=on  OutDataTypeStr=Inherit: Same as first input
  RAPdot=RAPdel/AffTau1 : Product  Inputs=/*  SaturateOnIntegerOverflow=on  InputSameDT=on  OutDataTypeStr=Inherit: Same as first input
  RAPdot=RAPdel/AffTau2 : Product  SaturateOnIntegerOverflow=on  InputSameDT=on  OutDataTypeStr=Inherit: Same as first input
  RAPdot=RAPdel/AffTau3 : Product  Inputs=/*  SaturateOnIntegerOverflow=on  InputSameDT=on  OutDataTypeStr=Inherit: Same as first input
  SR : Constant
  SR2 : Constant  Value=8
  SRK2 : Constant  Value=10000
  VV6init : Constant  Value=0
  VV7init : Constant  Value=0
  VV6 : Outport
  VV7 : Outport  Port=2
  wires:
  ISRK1/1 -> RAPdot=RAPdel/AffTau3/1
  RAPdot=RAPdel/AffTau3/1 -> Integrator2/1
  RAPDel=RAP-RAPAdp2/1 -> RAPdot=RAPdel/AffTau3/2
  VV7init/1 -> Integrator2/2
  VV6init/1 -> Integrator1/2
  Integrator2/1 -> RAPDel=RAP-RAPAdp2/2, VV7/1  "VV7"
  RAPdot=RAPdel/AffTau2/1 -> RAPDel=RAP-RAPAdp2/1
  SR/1 -> RAPdot=RAPdel/AffTau2/2
  RAPdot=RAPdel/AffTau1/1 -> Integrator1/1
  RAPDel=RAP-RAPAdp1/1 -> RAPdot=RAPdel/AffTau1/2
  SRK2/1 -> RAPdot=RAPdel/AffTau1/1
  RAPdot=RAPdel/AffTau/1 -> RAPDel=RAP-RAPAdp1/1
  SR2/1 -> RAPdot=RAPdel/AffTau/1
  RAPDel=RAP-RAPAdp/1 -> RAPdot=RAPdel/AffTau2/1, RAPdot=RAPdel/AffTau/2
  VVE/1 -> RAPDel=RAP-RAPAdp/1
  " 2"/1 -> RAPDel=RAP-RAPAdp/2
  Integrator1/1 -> VV6/1, RAPDel=RAP-RAPAdp1/2  "VV6"

== system GuytonModel1986All_R2015a/Efferent Arteriole ==
  note: EFFERENT ARTERIOLE
  EARK : Inport
  RNAUG1 : Inport  Port=2
  EFARF : Inport  Port=3
  ANM : Inport  Port=4
  VIM : Inport  Port=5
  ANMAM1 : Constant
  ANMEM : Constant  Value=1.5
  Constant1 : Constant
  Constant2 : Constant
  Constant35 : Constant
  Product11 : Product  SaturateOnIntegerOverflow=on  RndMeth=Zero  InputSameDT=on  OutDataTypeStr=Inherit: Same as first input
  Product12 : Product  Inputs=4  SaturateOnIntegerOverflow=on  RndMeth=Zero  InputSameDT=on  OutDataTypeStr=Inherit: Same as first input
  Product2 : Product  SaturateOnIntegerOverflow=on  RndMeth=Zero  InputSameDT=on  OutDataTypeStr=Inherit: Same as first input
  Sum1 : Sum  SaturateOnIntegerOverflow=on  InputSameDT=on  OutDataTypeStr=Inherit: Same as first input
  Sum18 : Sum  Inputs=+-  SaturateOnIntegerOverflow=on  InputSameDT=on  OutDataTypeStr=Inherit: Same as first input
  Sum2 : Sum  SaturateOnIntegerOverflow=on  InputSameDT=on  OutDataTypeStr=Inherit: Same as first input
  Sum4 : Sum  Inputs=+-  SaturateOnIntegerOverflow=on  InputSameDT=on  OutDataTypeStr=Inherit: Same as first input
  lower limit 0.86 : Saturate  UpperLimit=inf  LowerLimit=0.86
  lower limit 24 : Saturate  UpperLimit=inf  LowerLimit=24
  EAR : Outport
  wires:
  ANM/1 -> Sum18/1
  Constant35/1 -> Sum18/2
  ANMEM/1 -> Product11/2
  Sum18/1 -> Product11/1
  Product12/1 -> lower limit 24/1
  lower limit 24/1 -> EAR/1
  Product11/1 -> Sum1/1
  ANMAM1/1 -> Sum1/2
  Sum1/1 -> lower limit 0.86/1
  EARK/1 -> Product12/1  "EARK"
  RNAUG1/1 -> Sum4/1
  Sum4/1 -> Product2/1
  EFARF/1 -> Product2/2
  VIM/1 -> Product12/2  "VIM"
  Constant2/1 -> Sum4/2
  lower limit 0.86/1 -> Product12/4  "ANMER"
  Product2/1 -> Sum2/2
  Sum2/1 -> Product12/3  "MDEA"
  Constant1/1 -> Sum2/1

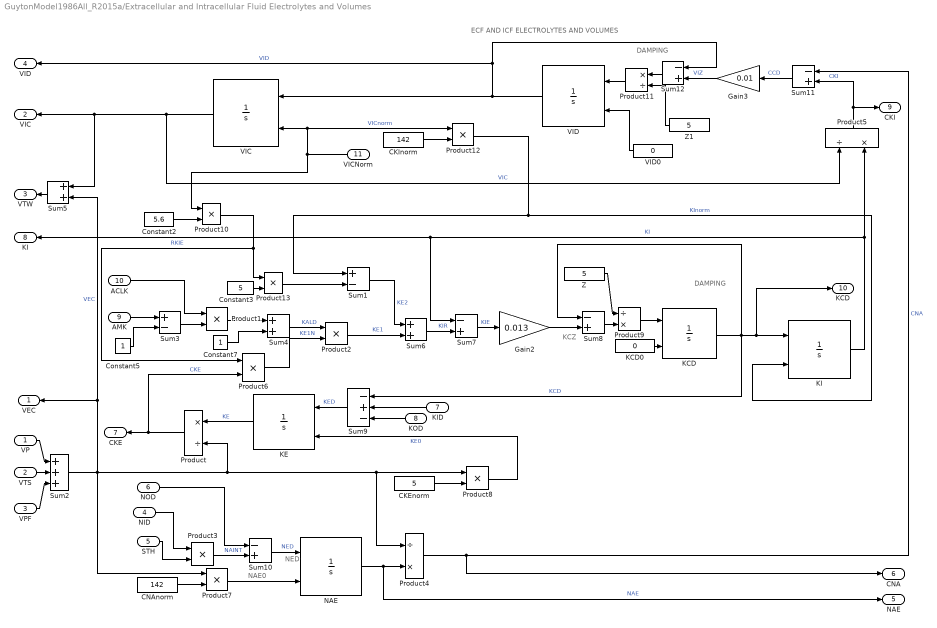
== system GuytonModel1986All_R2015a/Extracellular and Intracellular Fluid Electrolytes and Volumes ==
  note: ECF AND ICF ELECTROLYTES AND VOLUMES
  note: DAMPING
  note: KCZ
  note: NAE0
  note: NED
  note: DAMPING
  VP : Inport
  VTS : Inport  Port=2
  VPF : Inport  Port=3
  NID : Inport  Port=4
  STH : Inport  Port=5
  NOD : Inport  Port=6
  KID : Inport  Port=7
  KOD : Inport  Port=8
  AMK : Inport  Port=9
  ACLK : Inport  Port=10
  VICNorm : Inport  Port=11
  CKEnorm : Constant  Value=5
  CKInorm : Constant  Value=142
  CNAnorm : Constant  Value=142
  Constant2 : Constant  Value=5.6
  Constant3 : Constant  Value=5
  Constant5 : Constant
  Constant7 : Constant
  Gain2 : Gain  Gain=0.013  SaturateOnIntegerOverflow=on  OutDataTypeStr=Inherit: Same as input  ParamDataTypeStr=Inherit: Same as input
  Gain3 : Gain  Gain=0.01  SaturateOnIntegerOverflow=on  OutDataTypeStr=Inherit: Same as input  ParamDataTypeStr=Inherit: Same as input
  "KCD " : Integrator  InitialConditionSource=external  InitialCondition=0.000024999
  KCD0 : Constant  Value=0
  "KE " : Integrator  InitialConditionSource=external  InitialCondition=74.7024
  "KI " : Integrator  InitialConditionSource=external  InitialCondition=3549.44848
  "NAE " : Integrator  InitialConditionSource=external  InitialCondition=2120.8784
  Product : Product  Inputs=*/  SaturateOnIntegerOverflow=on  RndMeth=Zero  InputSameDT=on  OutDataTypeStr=Inherit: Same as first input
  Product{1..3,6..8,10,12..13} (9 alike) : Product  SaturateOnIntegerOverflow=on  RndMeth=Zero  InputSameDT=on  OutDataTypeStr=Inherit: Same as first input
  Product11 : Product  Inputs=*/  SaturateOnIntegerOverflow=on  RndMeth=Zero  InputSameDT=on  OutDataTypeStr=Inherit: Same as first input
  Product4 : Product  Inputs=/*  SaturateOnIntegerOverflow=on  RndMeth=Zero  InputSameDT=on  OutDataTypeStr=Inherit: Same as first input
  Product5 : Product  Inputs=/*  SaturateOnIntegerOverflow=on  RndMeth=Zero  InputSameDT=on  OutDataTypeStr=Inherit: Same as first input
  Product9 : Product  Inputs=/*  SaturateOnIntegerOverflow=on  RndMeth=Zero  InputSameDT=on  OutDataTypeStr=Inherit: Same as first input
  Sum1 : Sum  Inputs=+-  SaturateOnIntegerOverflow=on  InputSameDT=on  OutDataTypeStr=Inherit: Same as first input
  Sum{7..8,10..12} (5 alike) : Sum  Inputs=-+  SaturateOnIntegerOverflow=on  InputSameDT=on  OutDataTypeStr=Inherit: Same as first input
  Sum2 : Sum  Inputs=+++  SaturateOnIntegerOverflow=on  InputSameDT=on  OutDataTypeStr=Inherit: Same as first input
  Sum3 : Sum  Inputs=+-  SaturateOnIntegerOverflow=on  InputSameDT=on  OutDataTypeStr=Inherit: Same as first input
  Sum4 : Sum  SaturateOnIntegerOverflow=on  InputSameDT=on  OutDataTypeStr=Inherit: Same as first input
  Sum5 : Sum  SaturateOnIntegerOverflow=on  InputSameDT=on  OutDataTypeStr=Inherit: Same as first input
  Sum6 : Sum  SaturateOnIntegerOverflow=on  InputSameDT=on  OutDataTypeStr=Inherit: Same as first input
  Sum9 : Sum  Inputs=-+-  SaturateOnIntegerOverflow=on  InputSameDT=on  OutDataTypeStr=Inherit: Same as first input
  "VIC " : Integrator  InitialConditionSource=external  InitialCondition=25.002477
  "VID " : Integrator  InitialConditionSource=external  InitialCondition=0.0000010839
  VID0 : Constant  Value=0
  Z : Constant  Value=5
  Z1 : Constant  Value=5
  VEC : Outport
  VIC : Outport  Port=2
  VTW : Outport  Port=3
  VID : Outport  Port=4
  NAE : Outport  Port=5
  CNA : Outport  Port=6
  CKE : Outport  Port=7
  KI : Outport  Port=8
  CKI : Outport  Port=9
  KCD : Outport  Port=10
  wires:
  Constant3/1 -> Product13/2
  Product10/1 -> Product6/1, Product13/1  "RKIE"
  Constant2/1 -> Product10/2
  Sum5/1 -> VTW/1
  "KCD "/1 -> Sum9/1, KCD/1, "KI "/1, Sum8/1  "KCD"
  "KI "/1 -> KI/1, Sum7/1, Product5/2  "KI"
  Z1/1 -> Product11/2
  VID0/1 -> "VID "/2
  KCD0/1 -> "KCD "/2
  Sum4/1 -> Product2/1  "KALD"
  Product6/1 -> Product2/2  "KE1N"
  Sum1/1 -> Sum6/1  "KE2"
  Product13/1 -> Sum1/2
  Product12/1 -> Sum1/1, "KI "/2  "KInorm"
  CKInorm/1 -> Product12/2
  VICNorm/1 -> Product10/1, "VIC "/2, Product12/1  "VICnorm"
  CKEnorm/1 -> Product8/2
  CNAnorm/1 -> Product7/2
  Product8/1 -> "KE "/2  "KE0"
  "NAE "/1 -> NAE/1, Product4/2  "NAE"
  Product7/1 -> "NAE "/2
  Sum2/1 -> Sum5/2, VEC/1, Product8/1, Product4/1, Product/2, Product7/1  "VEC"
  Product3/1 -> Sum10/2  "NAINT"
  STH/1 -> Product3/2
  NID/1 -> Product3/1
  NOD/1 -> Sum10/1
  KOD/1 -> Sum9/3
  KID/1 -> Sum9/2
  Product2/1 -> Sum6/2  "KE1"
  Product/1 -> Product6/2, CKE/1  "CKE"
  Constant7/1 -> Sum4/2
  Product1/1 -> Sum4/1
  ACLK/1 -> Product1/1
  Sum3/1 -> Product1/2
  Constant5/1 -> Sum3/2
  AMK/1 -> Sum3/1
  VPF/1 -> Sum2/3
  VP/1 -> Sum2/1
  VTS/1 -> Sum2/2
  Sum10/1 -> "NAE "/1  "NED"
  Product4/1 -> CNA/1, Sum11/1  "CNA"
  Sum9/1 -> "KE "/1  "KED"
  "KE "/1 -> Product/1  "KE"
  Sum8/1 -> Product9/2
  Product9/1 -> "KCD "/1
  "VIC "/1 -> VIC/1, Sum5/1, Product5/1  "VIC"
  Sum6/1 -> Sum7/2  "KIR"
  Sum7/1 -> Gain2/1  "KIE"
  Gain2/1 -> Sum8/2
  Product5/1 -> CKI/1, Sum11/2  "CKI"
  Sum11/1 -> Gain3/1  "CCD"
  Product11/1 -> "VID "/1
  Z/1 -> Product9/1
  "VID "/1 -> VID/1, Sum12/1, "VIC "/1  "VID"
  Sum12/1 -> Product11/1
  Gain3/1 -> Sum12/2  "VIZ"

== system GuytonModel1986All_R2015a/Glomerulus ==
  note: GLOMERULUS
  note: RPNIN
  note: GFN
  note: lower limit 0.001
  note: GFN
  PAR : Inport
  RFN : Inport  Port=2
  AAR : Inport  Port=3
  HM : Inport  Port=4
  PPC : Inport  Port=5
  PXTP : Inport  Port=6
  GLFC : Inport  Port=7
  REK : Inport  Port=8
  Constant1 : Constant  Value=0.98
  Constant2 : Constant  Value=1.35
  Constant3 : Constant  Value=37.929
  Constant4 : Constant  Value=0.123
  Constant45 : Constant
  GFNDMP : Constant  Value=3
  GPPD : Constant  Value=50
  Integrator1 : Integrator  InitialConditionSource=external
  Integrator2 : Integrator  InitialConditionSource=external  LimitOutput=on  LowerSaturationLimit=0.001
  Math Function1 : Math  Operator=pow  SaturateOnIntegerOverflow=on
  Product{1..2,4..5,7..8} (6 alike) : Product  SaturateOnIntegerOverflow=on  RndMeth=Zero  InputSameDT=on  OutDataTypeStr=Inherit: Same as first input
  Product3 : Product  Inputs=*/  SaturateOnIntegerOverflow=on  RndMeth=Zero  InputSameDT=on  OutDataTypeStr=Inherit: Same as first input
  Product6 : Product  Inputs=*/  SaturateOnIntegerOverflow=on  RndMeth=Zero  InputSameDT=on  OutDataTypeStr=Inherit: Same as first input
  Product9 : Product  Inputs=/*  SaturateOnIntegerOverflow=on  RndMeth=Zero  InputSameDT=on  OutDataTypeStr=Inherit: Same as first input
  Sum{1..2,4,6} (4 alike) : Sum  Inputs=+-  SaturateOnIntegerOverflow=on  InputSameDT=on  OutDataTypeStr=Inherit: Same as first input
  Sum3 : Sum  Inputs=-+  SaturateOnIntegerOverflow=on  InputSameDT=on  OutDataTypeStr=Inherit: Same as first input
  Sum5 : Sum  Inputs=--+  SaturateOnIntegerOverflow=on  InputSameDT=on  OutDataTypeStr=Inherit: Same as first input
  lower limit 1.0 : Saturate  UpperLimit=inf  LowerLimit=1  LinearizeAsGain=off
  GFR : Outport
  GFN : Outport  Port=2
  GLP : Outport  Port=3
  GLPC : Outport  Port=4
  PFL : Outport  Port=5
  wires:
  RFN/1 -> Product2/1, Product1/1
  Constant45/1 -> Sum1/1
  HM/1 -> Sum1/2
  Sum1/1 -> Product2/2
  Product2/1 -> Product3/1, Sum2/1
  Sum2/1 -> Product3/2  "RPNOUT"
  Product3/1 -> lower limit 1.0/1  "EFAFPR"
  lower limit 1.0/1 -> Product4/2
  Constant1/1 -> Product4/1
  Constant2/1 -> Math Function1/2
  Product4/1 -> Math Function1/1
  Math Function1/1 -> Product5/1
  PPC/1 -> Product5/2
  Constant3/1 -> Integrator1/2
  GPPD/1 -> Product6/2
  Product6/1 -> Integrator1/1  "DGLPC"
  Sum4/1 -> Product6/1
  Integrator1/1 -> Sum5/2, Sum4/2, GLPC/1  "GLPC"
  Product5/1 -> Sum4/1  "GLPC0"
  Product1/1 -> Sum3/1  "APD"
  AAR/1 -> Product1/2
  PAR/1 -> Sum3/2
  Sum3/1 -> Sum5/3, GLP/1  "GLP"
  PXTP/1 -> Sum5/1
  Sum5/1 -> Product7/2, PFL/1  "PFL"
  GLFC/1 -> Product7/1
  Constant4/1 -> Integrator2/2
  Product7/1 -> Sum6/1  "GFN0"
  Integrator2/1 -> Sum6/2, Sum2/2, Product8/2, GFN/1  "GFN"
  REK/1 -> Product8/1
  Product8/1 -> GFR/1
  Sum6/1 -> Product9/2
  Product9/1 -> Integrator2/1
  GFNDMP/1 -> Product9/1

== system GuytonModel1986All_R2015a/Heart Rate and Stroke Volume ==
  note: Heart Rate and Stroke Volume
  AUR : Inport
  HMD : Inport  Port=2
  PRA : Inport  Port=3
  QLO : Inport  Port=4
  " 1" : Constant  Value=32
  " 2" : Constant
  " 3" : Constant
  Divide1 : Product
  Divide2 : Product  Inputs=/*
  Gain : Gain  Gain=40
  Gain1 : Gain  Gain=2
  Gain2 : Gain  Gain=0.5
  Sum : Sum  Inputs=+++
  Sum1 : Sum  Inputs=+-
  Sum2 : Sum
  HR : Outport
  SVO : Outport  Port=2
  wires:
  Gain2/1 -> Sum2/2
  Divide2/1 -> SVO/1  "SVO"
  QLO/1 -> Divide2/2
  Divide1/1 -> Divide2/1, HR/1  "HR"
  Sum2/1 -> Divide1/2
  Sum/1 -> Divide1/1
  " 3"/1 -> Sum2/1
  Sum1/1 -> Gain2/1
  " 2"/1 -> Sum1/2
  HMD/1 -> Sum1/1
  " 1"/1 -> Sum/1
  Gain/1 -> Sum/2
  Gain1/1 -> Sum/3
  PRA/1 -> Gain1/1
  AUR/1 -> Gain/1

== system GuytonModel1986All_R2015a/Heart hypertrophy or deterioration ==
  note: 0<HMD<1
  note: HMD
  note: HPL
  note: HPR
  note: Heart hypertrophy or deterioration
  PA : Inport
  QAO : Inport  Port=2
  PPA : Inport  Port=3
  HSR : Inport  Port=4
  HSL : Inport  Port=5
  POT : Inport  Port=6
  Constant11 : Constant  Value=500
  Constant13 : Constant  Value=57600
  Constant15 : Constant  Value=75
  Constant17 : Constant  Value=57600
  Constant20 : Constant  Value=5
  Gain4 : Gain  Gain=0.0025  SaturateOnIntegerOverflow=on  OutDataTypeStr=Inherit: Same as input  ParamDataTypeStr=Inherit: Same as input
  "HMD " : Integrator  InitialConditionSource=external  InitialCondition=1  LimitOutput=on  UpperSaturationLimit=1  LowerSaturationLimit=0
  HMD0 : Constant
  HPL0 : Constant
  HPL1=PA4^Z13 : Math  Operator=pow  SaturateOnIntegerOverflow=on
  HPR0 : Constant
  HPR1=PP3^Z13 : Math  Operator=pow  SaturateOnIntegerOverflow=on
  Integrator1 : Integrator  InitialConditionSource=external  InitialCondition=1
  Integrator2 : Integrator  InitialConditionSource=external  InitialCondition=1
  Product{6..11} (6 alike) : Product  Inputs=*/  SaturateOnIntegerOverflow=on  RndMeth=Zero  InputSameDT=on  OutDataTypeStr=Inherit: Same as first input
  Product2 : Product  SaturateOnIntegerOverflow=on  RndMeth=Zero  InputSameDT=on  OutDataTypeStr=Inherit: Same as first input
  Product3 : Product  SaturateOnIntegerOverflow=on  RndMeth=Zero  InputSameDT=on  OutDataTypeStr=Inherit: Same as first input
  Sum5 : Sum  Inputs=+-  SaturateOnIntegerOverflow=on  InputSameDT=on  OutDataTypeStr=Inherit: Same as first input
  Sum6 : Sum  Inputs=+-  SaturateOnIntegerOverflow=on  InputSameDT=on  OutDataTypeStr=Inherit: Same as first input
  Sum7 : Sum  Inputs=+-  SaturateOnIntegerOverflow=on  InputSameDT=on  OutDataTypeStr=Inherit: Same as first input
  Z13 : Constant  Value=0.625
  lower limit = 0 : Saturate  UpperLimit=inf  LowerLimit=0
  lower limit = 1 : Saturate  UpperLimit=inf  LowerLimit=0
  HPR : Outport
  HPL : Outport  Port=2
  HMD : Outport  Port=3
  wires:
  Gain4/1 -> "HMD "/1
  HMD0/1 -> "HMD "/2
  HPR0/1 -> Integrator2/2
  Sum6/1 -> Product11/1
  HPR1=PP3^Z13/1 -> Sum6/1  "HPR1"
  HPL0/1 -> Integrator1/2
  POT/1 -> Sum7/1
  HSL/1 -> Product7/2
  HSR/1 -> Product10/2
  PPA/1 -> Product3/1
  QAO/1 -> Product3/2, Product2/2
  PA/1 -> Product2/1
  Sum7/1 -> Gain4/1
  Constant20/1 -> Sum7/2
  Product2/1 -> Product6/1
  Constant11/1 -> Product6/2
  Product6/1 -> Product7/1
  Constant13/1 -> Product8/2
  Product8/1 -> Integrator1/1
  Integrator1/1 -> HPL/1, Sum5/2  "HPL"
  Product3/1 -> Product9/1
  Constant15/1 -> Product9/2
  Product9/1 -> Product10/1
  Constant17/1 -> Product11/2
  Product11/1 -> Integrator2/1
  Integrator2/1 -> HPR/1, Sum6/2
  Z13/1 -> HPR1=PP3^Z13/2, HPL1=PA4^Z13/2
  HPL1=PA4^Z13/1 -> Sum5/1  "HPL1"
  Sum5/1 -> Product8/1
  "HMD "/1 -> HMD/1
  Product10/1 -> lower limit = 0/1  "PP3"
  lower limit = 0/1 -> HPR1=PP3^Z13/1
  Product7/1 -> lower limit = 1/1  "PA4"
  lower limit = 1/1 -> HPL1=PA4^Z13/1

== system GuytonModel1986All_R2015a/Interstitial Tissue Fluids, Pressures and Gel Dynamics ==
  note: CPI
  note: PLD1
  note: 2
      | PTCR=0.28*CPI+0.0019*CPI
  note: TPGHF
  note: 2
      | CHY=(HYL/VTS/5)
  note: 2
      | PTT=(VTS-VTSFI)/VTSFI)
  note: Interstitial Tissue Fluids, Pressures and Gel Dynamics
  VTS : Inport
  DPC : Inport  Port=2
  TSP0 : Inport  Port=3
  Add{,1..3,6..7} (6 alike) : Sum  Inputs=+-
  Add4 : Sum
  Add5 : Sum  Inputs=-++
  Constant1 : Constant  Value=0.28
  Constant2 : Constant  Value=0.0019
  Constant3 : Constant  Value=2
  Constant4 : Constant  Value=7
  Constant5 : Constant  Value=0.02
  Constant6 : Constant  Value=0
  Constant7 : Constant  Value=5
  GCOPF : Constant  Value=0.7
  HYL : Constant  Value=60
  Integrator1 : Integrator  InitialConditionSource=external
  Math Function : Math  Operator=square  SaturateOnIntegerOverflow=on
  Math Function1 : Math  Operator=square  SaturateOnIntegerOverflow=on
  Math Function2 : Math  Operator=square  SaturateOnIntegerOverflow=on
  PGHF : Constant  Value=3.7
  PLDF : Constant  Value=5.9
  Product : Product  Inputs=*/  RndMeth=Zero
  Product1 : Product  Inputs=*//  RndMeth=Zero
  Product{2..3,5..6,8..9} (6 alike) : Product  Inputs=**  RndMeth=Zero
  Product4 : Product  Inputs=/*  RndMeth=Zero
  Product7 : Product  Inputs=***  RndMeth=Zero
  VTSFI : Constant  Value=6
  function interstitialGelVolume(VTS) x=[0,12,15,18,21,24.0] y=[0,11.4,14.0,16.0,17.3,18.0] : Lookup_n-D  NumberOfTableDimensions=1  BreakpointsForDimension1=[0,12,15,18,21,24.0]  Table=[0,11.4,14.0,16.0,17.3,18.0]  InterpMethod=Cubic spline  ExtrapMethod=Clip  InputSameDT=on
  "if (PLD1>7)  {PLD=7} else {PLD=PLD1}" : Switch  Criteria=u2 > Threshold  Threshold=7
  "if (VTL1<0)  {VTL=0} else {VTL=VTL1}" : Switch
  PGH : Outport
  PTC : Outport  Port=2
  VTL : Outport  Port=3
  DPL : Outport  Port=4
  CPI : Outport  Port=5
  PTT : Outport  Port=6
  PIF : Outport  Port=7
  PTS : Outport  Port=8
  VIF : Outport  Port=9
  VG : Outport  Port=10
  TSP : Outport  Port=11
  wires:
  Integrator1/1 -> TSP/1, Product4/2  "TSP"
  TSP0/1 -> Integrator1/2
  DPC/1 -> Add7/1
  Add7/1 -> Integrator1/1
  Product9/1 -> DPL/1, Add7/2  "DPL"
  Product6/1 -> Add4/2
  Constant2/1 -> Product6/2
  Math Function2/1 -> Product6/1
  HYL/1 -> Product1/1
  Add6/1 -> PTS/1
  "if (VTL1<0)  {VTL=0} else {VTL=VTL1}"/1 -> Product9/2, VTL/1  "VTL"
  Constant6/1 -> "if (VTL1<0)  {VTL=0} else {VTL=VTL1}"/3
  Product8/1 -> "if (VTL1<0)  {VTL=0} else {VTL=VTL1}"/1, "if (VTL1<0)  {VTL=0} else {VTL=VTL1}"/2
  "if (PLD1>7)  {PLD=7} else {PLD=PLD1}"/1 -> Product8/2  "PLD"
  Constant5/1 -> Product8/1
  Constant4/1 -> "if (PLD1>7)  {PLD=7} else {PLD=PLD1}"/1
  Add5/1 -> "if (PLD1>7)  {PLD=7} else {PLD=PLD1}"/3, "if (PLD1>7)  {PLD=7} else {PLD=PLD1}"/2
  PLDF/1 -> Add5/2
  Product7/1 -> PTC/1
  GCOPF/1 -> Product7/3
  Add4/1 -> Product7/2  "PTCPR"
  Product5/1 -> Add4/1
  Constant1/1 -> Product5/1
  Product4/1 -> CPI/1, Product9/1, Math Function2/1, Product5/2
  Add3/1 -> Add6/2, PIF/1, Add5/3  "PIF"
  Add2/1 -> PGH/1, Add3/1  "PGH"
  Product3/1 -> Product7/1, Add3/2  "POSHYL"
  Constant3/1 -> Product3/2
  PGHF/1 -> Product2/1
  Product2/1 -> Add2/2
  Math Function1/1 -> Product3/1, Product2/2  "CHY"
  Product1/1 -> Math Function1/1
  Constant7/1 -> Product1/3
  VTSFI/1 -> Add1/2, Product/2
  Math Function/1 -> Add6/1, Add5/1, PTT/1, Add2/1  "PTT"
  Product/1 -> Math Function/1
  Add1/1 -> Product/1
  Add/1 -> VIF/1
  function interstitialGelVolume(VTS) x=[0,12,15,18,21,24.0] y=[0,11.4,14.0,16.0,17.3,18.0]/1 -> VG/1, Add/2  "VG"
  VTS/1 -> Add/1, Product1/2, Add1/1, Product4/1, function interstitialGelVolume(VTS) x=[0,12,15,18,21,24.0] y=[0,11.4,14.0,16.0,17.3,18.0]/1  "VTS"

== system GuytonModel1986All_R2015a/Left Heart Pumping ==
  note: Left Heart Pumping
  PLA : Inport
  PA : Inport  Port=2
  AUH : Inport  Port=3
  OSA : Inport  Port=4
  HSL : Inport  Port=5
  HPL : Inport  Port=6
  HMD : Inport  Port=7
  Display3 : Display
  Divide1 : Product  Inputs=**
  Divide2 : Product  Inputs=*/
  Divide3 : Product  Inputs=6
  function StarlingLNorm(PLA) cubic spline interpolation x=[-4.5,-4,0,-1,3,6,10] y=[0,0.01,3.6,5.05,9.4,11.6,13.5] : Lookup_n-D  NumberOfTableDimensions=1  BreakpointsForDimension1=[-10,-9,-8,-7,-6,-5,-4.5,-4, -1,0, 3, 6, 10,11,12,13,15]  Table=[0,0,0,0,0,0,0,0.01, 3.6,5.05, 9.4, 11.6,13.5, 13.5, 13.5, 13.5,13.5]  InterpMethod=Cubic spline  ExtrapMethod=Clip  InputSameDT=on
  "function leftHeartLoading(PA2) cubic spline interpolation x=[0,100, 125, 160, 200, 240] y=[1.04, 1.0,0.97,0.88,0.59,0]" : Lookup_n-D  NumberOfTableDimensions=1  BreakpointsForDimension1=[0,60,100, 125, 160, 200, 240]  Table=[1.04, 1.025,1,0.97,0.88,0.59,0]  InterpMethod=Cubic spline  ExtrapMethod=Clip  InputSameDT=on
  QLO : Outport
  QLN : Outport  Port=2
  LVM : Outport  Port=3
  wires:
  PA/1 -> Divide2/1
  HMD/1 -> Divide3/6
  HPL/1 -> Divide3/5
  HSL/1 -> Divide3/4
  Divide3/1 -> QLO/1  "QLO"
  AUH/1 -> Divide3/3, Divide1/2
  OSA/1 -> Divide1/1
  "function leftHeartLoading(PA2) cubic spline interpolation x=[0,100, 125, 160, 200, 240] y=[1.04, 1.0,0.97,0.88,0.59,0]"/1 -> LVM/1, Divide3/2  "LVM"
  Divide2/1 -> Display3/1, "function leftHeartLoading(PA2) cubic spline interpolation x=[0,100, 125, 160, 200, 240] y=[1.04, 1.0,0.97,0.88,0.59,0]"/1  "PA2"
  Divide1/1 -> Divide2/2
  function StarlingLNorm(PLA) cubic spline interpolation x=[-4.5,-4,0,-1,3,6,10] y=[0,0.01,3.6,5.05,9.4,11.6,13.5]/1 -> Divide3/1, QLN/1  "QLN"
  PLA/1 -> function StarlingLNorm(PLA) cubic spline interpolation x=[-4.5,-4,0,-1,3,6,10] y=[0,0.01,3.6,5.05,9.4,11.6,13.5]/1
